simulink model "comper_zero_2"  (R2021a)
settings: Solver=VariableStepAuto  StartTime=0.0  StopTime=10.0  RelTol=1e-3
libraries: simulink x3
settings Model: Creator=yasso  LastModifiedBy=yasso

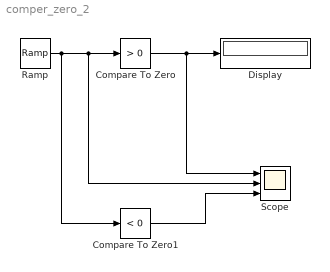
== system comper_zero_2 ==
  Compare To Zero : simulink/Logic and Bit Operations/Compare To Zero  relop=>  OutDataTypeStr=boolean
  Compare To Zero1 : simulink/Logic and Bit Operations/Compare To Zero  relop=<  OutDataTypeStr=boolean
  Display : Display
  Ramp : simulink/Sources/Ramp  slope=1  start=2  InitialOutput=-0.5
  Scope : Scope  NumInputPorts=3
  wires:
  Ramp/1 -> Compare To Zero1/1, Scope/2, Compare To Zero/1
  Compare To Zero/1 -> Scope/1, Display/1
  Compare To Zero1/1 -> Scope/3
